simulink model "sim_01"  (R2013a)
settings: Solver=ode4  StartTime=0.0  StopTime=StopTime  FixedStep=step  RelTol=1e-3
values from neighbouring files (symbols this model uses):
  mu = G*Mfix    (= 398571280000000)    [starter_sim_01.m]
  pos1_0 = [(6.371e+6+500) 0  0]    [starter_sim_01.m]
  pos2_0 = pos1_0+delta_pos1    [starter_sim_01.m]
  vel1_0 = [0 7.9e+3 4.5e+3]    [starter_sim_01.m]
  vel2_0 = vel1_0    [starter_sim_01.m]
undefined symbols (not defined in the file or in its folder): pos_0, vel_0
libraries: simulink x3, aerolibgravity2 x1
settings Model: Creator=enri  LastModifiedBy=enri

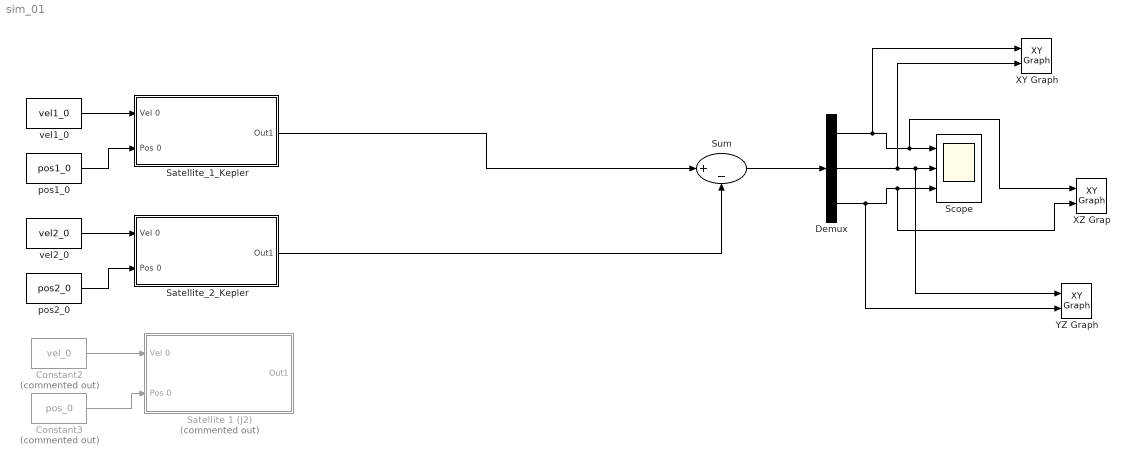
== system sim_01 ==
  Constant2 : Constant  Commented=on  Value=vel_0
  Constant3 : Constant  Commented=on  Value=pos_0
  Demux : Demux  Outputs=3
  Satellite 1 (J2) : Subsystem  Commented=on
  Satellite_1_Kepler : Subsystem
  Satellite_2_Kepler : Subsystem
  Scope : Scope  NumInputPorts=3
      settings: YMin=-5~-5~-5  YMax=5~5~5
  Sum : Sum  Inputs=|+-
  XY Graph : simulink/Sinks/XY Graph  xmin=-100000  xmax=100000  ymin=-100000  ymax=100000  st=-1
  XZ Grap : simulink/Sinks/XY Graph  xmin=-1  xmax=1  ymin=-1  ymax=1  st=-1
  YZ Graph : simulink/Sinks/XY Graph  xmin=-1  xmax=1  ymin=-1  ymax=1  st=-1
  pos1_0 : Constant  Value=pos1_0
  pos2_0 : Constant  Value=pos2_0
  vel1_0 : Constant  Value=vel1_0
  vel2_0 : Constant  Value=vel2_0
  wires:
  Sum/1 -> Demux/1
  Demux/2 -> XY Graph/2, YZ Graph/1, Scope/2
  Demux/3 -> YZ Graph/2, XZ Grap/2, Scope/3
  vel1_0/1 -> Satellite_1_Kepler/1(Vel 0)
  pos1_0/1 -> Satellite_1_Kepler/2(Pos 0)
  Constant2/1 -> Satellite 1 (J2)/1(Vel 0)
  Constant3/1 -> Satellite 1 (J2)/2(Pos 0)
  vel2_0/1 -> Satellite_2_Kepler/1(Vel 0)
  pos2_0/1 -> Satellite_2_Kepler/2(Pos 0)
  Satellite_2_Kepler/1(Out1) -> Sum/2
  Demux/1 -> XY Graph/1, XZ Grap/1, Scope/1
  Satellite_1_Kepler/1(Out1) -> Sum/1

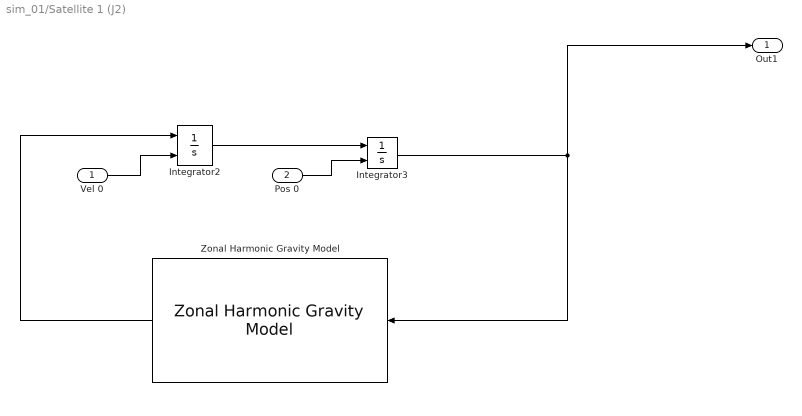
== system sim_01/Satellite 1 (J2) ==
  Vel 0 : Inport
  Pos 0 : Inport  Port=2
  Integrator2 : Integrator  InitialConditionSource=external
  Integrator3 : Integrator  InitialConditionSource=external  InitialCondition=pos_0
  Zonal Harmonic Gravity Model : aerolibgravity2/Zonal Harmonic Gravity Model  units=Metric (MKS)  degree=2  action=Warning  ptype=Earth  R=6378136.3  GM=398600441500000  jvalue=[1.0826269e-03 -2.5323000e-06 -1.6204000e-06]
  Out1 : Outport
  wires:
  Pos 0/1 -> Integrator3/2
  Zonal Harmonic Gravity Model/1 -> Integrator2/1
  Vel 0/1 -> Integrator2/2
  Integrator3/1 -> Out1/1, Zonal Harmonic Gravity Model/1
  Integrator2/1 -> Integrator3/1

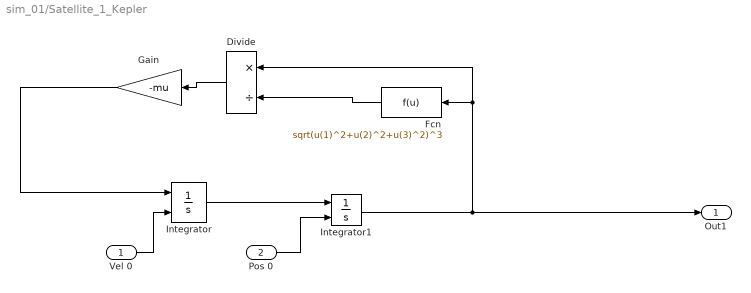
== system sim_01/Satellite_1_Kepler ==
  Vel 0 : Inport
  Pos 0 : Inport  Port=2
  Divide : Product  Inputs=*/
  Fcn : Fcn  Expr=sqrt(u(1)^2+u(2)^2+u(3)^2)^3
  Gain : Gain  Gain=-mu
  Integrator : Integrator  InitialConditionSource=external
  Integrator1 : Integrator  InitialConditionSource=external  InitialCondition=pos_0
  Out1 : Outport
  wires:
  Integrator/1 -> Integrator1/1
  Fcn/1 -> Divide/2
  Gain/1 -> Integrator/1
  Divide/1 -> Gain/1
  Pos 0/1 -> Integrator1/2
  Integrator1/1 -> Out1/1, Divide/1, Fcn/1
  Vel 0/1 -> Integrator/2

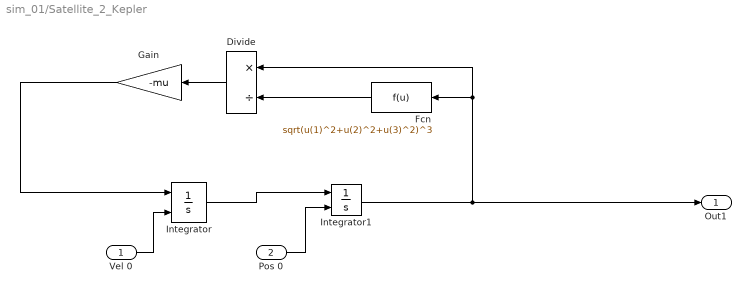
== system sim_01/Satellite_2_Kepler ==
  Vel 0 : Inport
  Pos 0 : Inport  Port=2
  Divide : Product  Inputs=*/
  Fcn : Fcn  Expr=sqrt(u(1)^2+u(2)^2+u(3)^2)^3
  Gain : Gain  Gain=-mu
  Integrator : Integrator  InitialConditionSource=external
  Integrator1 : Integrator  InitialConditionSource=external  InitialCondition=pos_0
  Out1 : Outport
  wires:
  Integrator/1 -> Integrator1/1
  Fcn/1 -> Divide/2
  Gain/1 -> Integrator/1
  Divide/1 -> Gain/1
  Pos 0/1 -> Integrator1/2
  Integrator1/1 -> Out1/1, Divide/1, Fcn/1
  Vel 0/1 -> Integrator/2
